simulink library "ddm"  (R2021b)
settings: Solver=VariableStepAuto  StartTime=0.0  StopTime=10.0  RelTol=1e-3
undefined symbols (not defined in the file or in its folder): ENUM_ADASACCSTA_ERROR, ENUM_ADASACCSTA_OFF, ENUM_ADASACCSTA_STANDBY, ENUM_ADASISASTA_OFF, ENUM_ALLOWMOV_ALLOWREADY, ENUM_APS, ENUM_BRKSTA_ERROR, ENUM_BRKSTA_OFF, ENUM_BRKSTA_ON, ENUM_BRKSW_INVALID, ENUM_BRKSW_OFF, ENUM_BRKSW_ON, ENUM_CHGPREACTERRSTA_OBCPRE, ENUM_DCDCFAULTSTA_ANYFAULTLV1, ENUM_DCDCFAULTSTA_ANYFAULTLV2, ENUM_DRIVETRAIN_AWD, ENUM_DRIVETRAIN_FWD, ENUM_DRIVETRAIN_RWD, ENUM_DRSEATSTA_INVALID, ENUM_EDUDRTSTA_NORMAL, ENUM_EPBSTA_APPLIED, ENUM_EPBSTA_RELEASED, ENUM_HVBATTREADYPRE_READY, ENUM_MCUWARN_LV0, ENUM_MCUWARN_LV1, ENUM_MCUWARN_LV2, ENUM_MCUWARN_LV3, ENUM_MCUWARN_NOERROR, ENUM_OBCFAULTSTA_ANYFAULT, ENUM_PAS_R2F2, ENUM_PDFAULT_BATTPDFAIL, ENUM_PDFAULT_DCDCDISABLE, ENUM_PDFAULT_MCUDISABLE, ENUM_PDFAULT_MCUDISCHRG, ENUM_POWERSTA_OFF, ENUM_POWERSTA_ON, ENUM_POWERSTA_READY, ENUM_POWERSTA_STANDBY, ENUM_PRESSINDI_LOW, ENUM_PUFAULT_BATTUPFAIL, ENUM_PUFAULT_DCDCENABLEFAIL, ENUM_PUFAULT_PRECHRGCHKFAIL, ENUM_PUFAULT_SAFETYCHKFAIL, ENUM_PUSTATE_COMPLETED, ENUM_PWRSTASW_OFF, ENUM_PWRSTASW_OFFA, ENUM_PWRSTASW_OFFCHVCHRG, ENUM_PWRSTASW_OFFCLVCHRG, ENUM_PWRSTASW_ON, ENUM_PWRSTASW_ONHVCHRG, ENUM_PWRSTASW_READY, ENUM_PWRSTASW_STANDBY, ENUM_RANGESTA_12IN, ENUM_SHIFTCOMMAND_D, ENUM_SHIFTCOMMAND_N, ENUM_SHIFTCOMMAND_P, ENUM_SHIFTCOMMAND_R, ENUM_VEHMALFUNLV_2ND, ENUM_VEHMALFUNLV_3RD, ENUM_VEHMALFUNLV_4TH ... (+835)
libraries: hcu_lib x750, $bdroot x12, simulink x5
(part 14 of 28)

== system ddm/DDM/DDM/VMC_DDM/CCU Signal Error ==
  task_time_s : Inport
  VDDM_C3CCU2LCCFS_flg : Inport  Port=2
  VDDM_C3CCU2RCCFS_flg : Inport  Port=3
  VDDM_C3CCU2CSCFS_flg : Inport  Port=4
  No_CAN_BUS_OFF : Inport  Port=5
  VPMM_PowerSta_enum : Inport  Port=6
  VINP_DCDCFaultSta_enum : Inport  Port=7
  DTC_clear_request : Inport  Port=8
  "CCU Signal Error " : Subsystem
  From5 : From  Commented=on  GotoTag=VDDM_CCUSigErrDFS_flg
  Terminator : Terminator
  VDDM_CCUSigErrCFS_flg : Outport
  VDDM_CCUSigErrDetDTC_raw32 : Outport  Port=2
  wires:
  [VDDM_CCUSigErrDetDTC_raw32] -> VDDM_CCUSigErrDetDTC_raw32/1
  "CCU Signal Error "/2(VDDM_CCUSigErrDetDTC_raw32) -> [VDDM_CCUSigErrDetDTC_raw32]
  [task_time_s] -> "CCU Signal Error "/1(task_time_s)
  task_time_s/1 -> [task_time_s]  "task_time_s"
  [DTC_clear_request] -> "CCU Signal Error "/8(DTC_clear_request)
  [VINP_DCDCFaultSta_enum] -> "CCU Signal Error "/7(VINP_DCDCFaultSta_enum)
  [VPMM_PowerSta_enum] -> "CCU Signal Error "/6(VPMM_PowerSta_enum)
  [No_CAN_BUS_OFF] -> "CCU Signal Error "/5(No_CAN_BUS_OFF)
  [VDDM_C3CCU2CSCFS_flg] -> "CCU Signal Error "/4(VDDM_C3CCU2CSCFS_flg)
  [VDDM_C3CCU2RCCFS_flg] -> "CCU Signal Error "/3(VDDM_C3CCU2RCCFS_flg)
  [VDDM_C3CCU2LCCFS_flg] -> "CCU Signal Error "/2(VDDM_C3CCU2LCCFS_flg)
  VINP_DCDCFaultSta_enum/1 -> [VINP_DCDCFaultSta_enum]
  VDDM_C3CCU2LCCFS_flg/1 -> [VDDM_C3CCU2LCCFS_flg]
  No_CAN_BUS_OFF/1 -> [No_CAN_BUS_OFF]
  VPMM_PowerSta_enum/1 -> [VPMM_PowerSta_enum]
  DTC_clear_request/1 -> [DTC_clear_request]
  "CCU Signal Error "/1(VDDM_CCUSigErrCFS_flg) -> [VDDM_CCUSigErrCFS_flg]
  From5/1 -> Terminator/1
  [VDDM_CCUSigErrCFS_flg] -> VDDM_CCUSigErrCFS_flg/1
  VDDM_C3CCU2RCCFS_flg/1 -> [VDDM_C3CCU2RCCFS_flg]
  VDDM_C3CCU2CSCFS_flg/1 -> [VDDM_C3CCU2CSCFS_flg]

== system ddm/DDM/DDM/VMC_DDM/FCM2 ==
  task_time_s : Inport
  VDDM_FCM2NoCom_flg : Inport  Port=2
  VDDM_FCM2RCErr_flg : Inport  Port=3
  VDDM_FCM2CSErr_flg : Inport  Port=4
  No_CAN_BUS_OFF : Inport  Port=5
  VPMM_PowerSta_enum : Inport  Port=6
  VINP_ADASACCSta_enum : Inport  Port=7
  DTC_clear_request : Inport  Port=8
  Constant18 : Constant  Commented=on  Value=TRUE
  Constant21 : Constant  Commented=on  Value=FALSE
  "FCM2 Checksum Error " : Subsystem
  FCM2 Lost Com : Subsystem
  "FCM2 Rolling Count Error " : Subsystem
  From15 : From  Commented=on  GotoTag=VDDM_FCM2NoComCFS_flg
  From16 : From  Commented=on  GotoTag=VDDM_FCM2RCErrCFS_flg
  From17 : From  Commented=on  GotoTag=VDDM_FCM2CSErrCFS_flg
  From30 : From  Commented=on  GotoTag=VDDM_VCUACCErr_flg
  Goto11 : Goto  Commented=on  GotoTag=VDDM_VCUACCErr_flg
  Logical Operator2 : Logic  Commented=on  Operator=OR  Inputs=3  AllPortsSameDT=off  OutDataTypeStr=boolean
  Switch : Switch  Commented=on  Criteria=u2 ~= 0
  Terminator : Terminator
  VDDM_FCM2NoComDFS_flg : Outport
  VDDM_FCM2NoComCFS_flg : Outport  Port=2
  VDDM_FCM2RCErrDFS_flg : Outport  Port=3
  VDDM_FCM2RCErrCFS_flg : Outport  Port=4
  VDDM_FCM2CSErrDFS_flg : Outport  Port=5
  VDDM_FCM2CSErrCFS_flg : Outport  Port=6
  VDDM_FCM2NoComDTC_raw32 : Outport  Port=7
  VDDM_FCM2RCErrDTC_raw32 : Outport  Port=8
  VDDM_FCM2CSErrDTC_raw32 : Outport  Port=9
  wires:
  [VDDM_FCM2CSErrDTC_raw32] -> VDDM_FCM2CSErrDTC_raw32/1
  [VDDM_FCM2RCErrDTC_raw32] -> VDDM_FCM2RCErrDTC_raw32/1
  [VDDM_FCM2NoComDTC_raw32] -> VDDM_FCM2NoComDTC_raw32/1
  "FCM2 Checksum Error "/3(VDDM_FCM2CSErrDTC_raw32) -> [VDDM_FCM2CSErrDTC_raw32]
  "FCM2 Rolling Count Error "/3(VDDM_FCM2RCErrDTC_raw32) -> [VDDM_FCM2RCErrDTC_raw32]
  FCM2 Lost Com/3(VDDM_FCM2NoComDTC_raw32) -> [VDDM_FCM2NoComDTC_raw32]
  "FCM2 Checksum Error "/2(VDDM_FCM2CSErrCFS_flg) -> [VDDM_FCM2CSErrCFS_flg]
  "FCM2 Checksum Error "/1(VDDM_FCM2CSErrDFS_flg) -> [VDDM_FCM2CSErrDFS_flg]
  [VDDM_FCM2NoComCFS_flg] -> "FCM2 Checksum Error "/4(VDDM_FCM2NoComCFS_flg)
  [VDDM_FCM2CSErr_flg] -> "FCM2 Checksum Error "/2(VDDM_FCM2CSErr_flg)
  [No_CAN_BUS_OFF] -> "FCM2 Checksum Error "/3(No_CAN_BUS_OFF)
  [VPMM_PowerSta_enum] -> "FCM2 Checksum Error "/5(VPMM_PowerSta_enum)
  [VINP_ADASACCSta_enum] -> "FCM2 Checksum Error "/6(VINP_ADASACCSta_enum)
  [DTC_clear_request] -> "FCM2 Checksum Error "/7(DTC_clear_request)
  [task_time_s] -> "FCM2 Checksum Error "/1(task_time_s)
  [task_time_s] -> "FCM2 Rolling Count Error "/1(task_time_s)
  task_time_s/1 -> [task_time_s]  "task_time_s"
  [task_time_s] -> FCM2 Lost Com/1(task_time_s)
  Logical Operator2/1 -> Switch/2
  From17/1 -> Logical Operator2/3
  From16/1 -> Logical Operator2/2
  From15/1 -> Logical Operator2/1
  Constant21/1 -> Switch/3
  Constant18/1 -> Switch/1
  VDDM_FCM2CSErr_flg/1 -> [VDDM_FCM2CSErr_flg]
  VDDM_FCM2RCErr_flg/1 -> [VDDM_FCM2RCErr_flg]
  From30/1 -> Terminator/1
  Switch/1 -> Goto11/1
  [VDDM_FCM2RCErrDFS_flg] -> VDDM_FCM2RCErrDFS_flg/1
  [VDDM_FCM2RCErrCFS_flg] -> VDDM_FCM2RCErrCFS_flg/1
  [VDDM_FCM2CSErrCFS_flg] -> VDDM_FCM2CSErrCFS_flg/1
  [VDDM_FCM2CSErrDFS_flg] -> VDDM_FCM2CSErrDFS_flg/1
  [VDDM_FCM2NoComCFS_flg] -> VDDM_FCM2NoComCFS_flg/1
  "FCM2 Rolling Count Error "/2(VDDM_FCM2RCErrCFS_flg) -> [VDDM_FCM2RCErrCFS_flg]
  "FCM2 Rolling Count Error "/1(VDDM_FCM2RCErrDFS_flg) -> [VDDM_FCM2RCErrDFS_flg]
  [DTC_clear_request] -> "FCM2 Rolling Count Error "/7(DTC_clear_request)
  [VINP_ADASACCSta_enum] -> "FCM2 Rolling Count Error "/6(VINP_ADASACCSta_enum)
  [VPMM_PowerSta_enum] -> "FCM2 Rolling Count Error "/5(VPMM_PowerSta_enum)
  [No_CAN_BUS_OFF] -> "FCM2 Rolling Count Error "/3(No_CAN_BUS_OFF)
  [VDDM_FCM2RCErr_flg] -> "FCM2 Rolling Count Error "/2(VDDM_FCM2RCErr_flg)
  [VDDM_FCM2NoComCFS_flg] -> "FCM2 Rolling Count Error "/4(VDDM_FCM2NoComCFS_flg)
  [VDDM_FCM2NoComDFS_flg] -> VDDM_FCM2NoComDFS_flg/1
  FCM2 Lost Com/1(VDDM_FCM2NoComDFS_flg) -> [VDDM_FCM2NoComDFS_flg]
  FCM2 Lost Com/2(VDDM_FCM2NoComCFS_flg) -> [VDDM_FCM2NoComCFS_flg]
  [DTC_clear_request] -> FCM2 Lost Com/6(DTC_clear_request)
  [VINP_ADASACCSta_enum] -> FCM2 Lost Com/5(VINP_ADASACCSta_enum)
  [VPMM_PowerSta_enum] -> FCM2 Lost Com/4(VPMM_PowerSta_enum)
  [No_CAN_BUS_OFF] -> FCM2 Lost Com/3(No_CAN_BUS_OFF)
  DTC_clear_request/1 -> [DTC_clear_request]
  VINP_ADASACCSta_enum/1 -> [VINP_ADASACCSta_enum]
  VPMM_PowerSta_enum/1 -> [VPMM_PowerSta_enum]
  No_CAN_BUS_OFF/1 -> [No_CAN_BUS_OFF]
  [VDDM_FCM2NoCom_flg] -> FCM2 Lost Com/2(VDDM_FCM2NoCom_flg)
  VDDM_FCM2NoCom_flg/1 -> [VDDM_FCM2NoCom_flg]

== system ddm/DDM/DDM/VMC_DDM/FCM3 ==
  task_time_s : Inport
  VDDM_FCM3NoCom_flg : Inport  Port=2
  VDDM_FCM3RCErr_flg : Inport  Port=3
  VDDM_FCM3CSErr_flg : Inport  Port=4
  No_CAN_BUS_OFF : Inport  Port=5
  VPMM_PowerSta_enum : Inport  Port=6
  VINP_ADASACCSta_enum : Inport  Port=7
  VINP_ADASISASta_enum : Inport  Port=8
  DTC_clear_request : Inport  Port=9
  Constant18 : Constant  Commented=on  Value=TRUE
  Constant21 : Constant  Commented=on  Value=FALSE
  "FCM3 Checksum Error " : Subsystem
  FCM3 Lost Com : Subsystem
  "FCM3 Rolling Count Error " : Subsystem
  From15 : From  Commented=on  GotoTag=VDDM_FCM3NoComCFS_flg
  From16 : From  Commented=on  GotoTag=VDDM_FCM3RCErrCFS_flg
  From17 : From  Commented=on  GotoTag=VDDM_FCM3CSErrCFS_flg
  From23 : From  Commented=on  GotoTag=VDDM_VCUISAErr_flg
  Goto11 : Goto  Commented=on  GotoTag=VDDM_VCUISAErr_flg
  Logical Operator2 : Logic  Commented=on  Operator=OR  Inputs=3  AllPortsSameDT=off  OutDataTypeStr=boolean
  Switch : Switch  Commented=on  Criteria=u2 ~= 0
  Terminator : Terminator
  VDDM_FCM3NoComDFS_flg : Outport
  VDDM_FCM3NoComCFS_flg : Outport  Port=2
  VDDM_FCM3RCErrDFS_flg : Outport  Port=3
  VDDM_FCM3RCErrCFS_flg : Outport  Port=4
  VDDM_FCM3CSErrDFS_flg : Outport  Port=5
  VDDM_FCM3CSErrCFS_flg : Outport  Port=6
  VDDM_FCM3NoComDTC_raw32 : Outport  Port=7
  VDDM_FCM3RCErrDTC_raw32 : Outport  Port=8
  VDDM_FCM3CSErrDTC_raw32 : Outport  Port=9
  wires:
  [VDDM_FCM3CSErrDTC_raw32] -> VDDM_FCM3CSErrDTC_raw32/1
  [VDDM_FCM3RCErrDTC_raw32] -> VDDM_FCM3RCErrDTC_raw32/1
  [VDDM_FCM3NoComDTC_raw32] -> VDDM_FCM3NoComDTC_raw32/1
  "FCM3 Checksum Error "/3(VDDM_FCM3CSErrDTC_raw32) -> [VDDM_FCM3CSErrDTC_raw32]
  "FCM3 Rolling Count Error "/3(VDDM_FCM3RCErrDTC_raw32) -> [VDDM_FCM3RCErrDTC_raw32]
  FCM3 Lost Com/3(VDDM_FCM3NoComDTC_raw32) -> [VDDM_FCM3NoComDTC_raw32]
  [VINP_ADASISASta_enum] -> "FCM3 Checksum Error "/7(VINP_ADASISASta_enum)
  [VINP_ADASISASta_enum] -> "FCM3 Rolling Count Error "/7(VINP_ADASISASta_enum)
  VINP_ADASISASta_enum/1 -> [VINP_ADASISASta_enum]
  [VINP_ADASISASta_enum] -> FCM3 Lost Com/6(VINP_ADASISASta_enum)
  "FCM3 Checksum Error "/2(VDDM_FCM3CSErrCFS_flg) -> [VDDM_FCM3CSErrCFS_flg]
  "FCM3 Checksum Error "/1(VDDM_FCM3CSErrDFS_flg) -> [VDDM_FCM3CSErrDFS_flg]
  [VDDM_FCM3NoComCFS_flg] -> "FCM3 Checksum Error "/4(VDDM_FCM3NoComCFS_flg)
  [VDDM_FCM3CSErr_flg] -> "FCM3 Checksum Error "/2(VDDM_FCM3CSErr_flg)
  [No_CAN_BUS_OFF] -> "FCM3 Checksum Error "/3(No_CAN_BUS_OFF)
  [VPMM_PowerSta_enum] -> "FCM3 Checksum Error "/5(VPMM_PowerSta_enum)
  [VINP_ADASACCSta_enum] -> "FCM3 Checksum Error "/6(VINP_ADASACCSta_enum)
  [DTC_clear_request] -> "FCM3 Checksum Error "/8(DTC_clear_request)
  [task_time_s] -> "FCM3 Checksum Error "/1(task_time_s)
  [task_time_s] -> "FCM3 Rolling Count Error "/1(task_time_s)
  task_time_s/1 -> [task_time_s]  "task_time_s"
  [task_time_s] -> FCM3 Lost Com/1(task_time_s)
  Logical Operator2/1 -> Switch/2
  From17/1 -> Logical Operator2/3
  From16/1 -> Logical Operator2/2
  From15/1 -> Logical Operator2/1
  Constant21/1 -> Switch/3
  Constant18/1 -> Switch/1
  VDDM_FCM3CSErr_flg/1 -> [VDDM_FCM3CSErr_flg]
  VDDM_FCM3RCErr_flg/1 -> [VDDM_FCM3RCErr_flg]
  From23/1 -> Terminator/1
  Switch/1 -> Goto11/1
  [VDDM_FCM3RCErrDFS_flg] -> VDDM_FCM3RCErrDFS_flg/1
  [VDDM_FCM3RCErrCFS_flg] -> VDDM_FCM3RCErrCFS_flg/1
  [VDDM_FCM3CSErrCFS_flg] -> VDDM_FCM3CSErrCFS_flg/1
  [VDDM_FCM3CSErrDFS_flg] -> VDDM_FCM3CSErrDFS_flg/1
  [VDDM_FCM3NoComCFS_flg] -> VDDM_FCM3NoComCFS_flg/1
  "FCM3 Rolling Count Error "/2(VDDM_FCM3RCErrCFS_flg) -> [VDDM_FCM3RCErrCFS_flg]
  "FCM3 Rolling Count Error "/1(VDDM_FCM3RCErrDFS_flg) -> [VDDM_FCM3RCErrDFS_flg]
  [DTC_clear_request] -> "FCM3 Rolling Count Error "/8(DTC_clear_request)
  [VINP_ADASACCSta_enum] -> "FCM3 Rolling Count Error "/6(VINP_ADASACCSta_enum)
  [VPMM_PowerSta_enum] -> "FCM3 Rolling Count Error "/5(VPMM_PowerSta_enum)
  [No_CAN_BUS_OFF] -> "FCM3 Rolling Count Error "/3(No_CAN_BUS_OFF)
  [VDDM_FCM3RCErr_flg] -> "FCM3 Rolling Count Error "/2(VDDM_FCM3RCErr_flg)
  [VDDM_FCM3NoComCFS_flg] -> "FCM3 Rolling Count Error "/4(VDDM_FCM3NoComCFS_flg)
  [VDDM_FCM3NoComDFS_flg] -> VDDM_FCM3NoComDFS_flg/1
  FCM3 Lost Com/1(VDDM_FCM3NoComDFS_flg) -> [VDDM_FCM3NoComDFS_flg]
  FCM3 Lost Com/2(VDDM_FCM3NoComCFS_flg) -> [VDDM_FCM3NoComCFS_flg]
  [DTC_clear_request] -> FCM3 Lost Com/7(DTC_clear_request)
  [VINP_ADASACCSta_enum] -> FCM3 Lost Com/5(VINP_ADASACCSta_enum)
  [VPMM_PowerSta_enum] -> FCM3 Lost Com/4(VPMM_PowerSta_enum)
  [No_CAN_BUS_OFF] -> FCM3 Lost Com/3(No_CAN_BUS_OFF)
  DTC_clear_request/1 -> [DTC_clear_request]
  VINP_ADASACCSta_enum/1 -> [VINP_ADASACCSta_enum]
  VPMM_PowerSta_enum/1 -> [VPMM_PowerSta_enum]
  No_CAN_BUS_OFF/1 -> [No_CAN_BUS_OFF]
  [VDDM_FCM3NoCom_flg] -> FCM3 Lost Com/2(VDDM_FCM3NoCom_flg)
  VDDM_FCM3NoCom_flg/1 -> [VDDM_FCM3NoCom_flg]

== system ddm/DDM/DDM/VMC_DDM/FCM4 ==
  task_time_s : Inport
  VDDM_FCM4NoCom_flg : Inport  Port=2
  VDDM_FCM4CSErr_flg : Inport  Port=3
  No_CAN_BUS_OFF : Inport  Port=4
  VPMM_PowerSta_enum : Inport  Port=5
  VINP_ADASACCSta_enum : Inport  Port=6
  DTC_clear_request : Inport  Port=7
  Constant18 : Constant  Commented=on  Value=TRUE
  Constant21 : Constant  Commented=on  Value=FALSE
  "FCM4 Checksum Error " : Subsystem
  FCM4 Lost Com : Subsystem
  "FCM4 Rolling Count Error " : Subsystem  Commented=on
  From10 : From  Commented=on  GotoTag=VINP_ADASACCSta_enum
  From11 : From  Commented=on  GotoTag=DTC_clear_request
  From15 : From  Commented=on  GotoTag=VDDM_FCM4NoComCFS_flg
  From16 : From  Commented=on  GotoTag=VDDM_FCM4RCErrCFS_flg
  From17 : From  Commented=on  GotoTag=VDDM_FCM4CSErrCFS_flg
  From19 : From  Commented=on  GotoTag=task_time_s
  From21 : From  Commented=on  GotoTag=VDDM_FCM4RCErrCFS_flg
  From22 : From  Commented=on  GotoTag=VDDM_FCM4RCErrDFS_flg
  From30 : From  Commented=on  GotoTag=VDDM_VCUACCErr_flg
  From6 : From  Commented=on  GotoTag=VDDM_FCM4NoComCFS_flg
  From7 : From  Commented=on  GotoTag=VDDM_FCM4RCErr_flg
  From8 : From  Commented=on  GotoTag=No_CAN_BUS_OFF
  From9 : From  Commented=on  GotoTag=VPMM_PowerSta_enum
  Goto11 : Goto  Commented=on  GotoTag=VDDM_VCUACCErr_flg
  Goto12 : Goto  Commented=on  GotoTag=VDDM_FCM4RCErr_flg
  Goto7 : Goto  Commented=on  GotoTag=VDDM_FCM4RCErrCFS_flg
  Goto8 : Goto  Commented=on  GotoTag=VDDM_FCM4RCErrDFS_flg
  Ground : Ground
  Logical Operator2 : Logic  Commented=on  Operator=OR  Inputs=3  AllPortsSameDT=off  OutDataTypeStr=boolean
  Switch : Switch  Commented=on  Criteria=u2 ~= 0
  Terminator : Terminator
  Terminator1 : Terminator
  Terminator2 : Terminator
  VDDM_FCM4NoComDFS_flg : Outport
  VDDM_FCM4NoComCFS_flg : Outport  Port=2
  VDDM_FCM4CSErrDFS_flg : Outport  Port=3
  VDDM_FCM4CSErrCFS_flg : Outport  Port=4
  VDDM_FCM4NoComDTC_raw32 : Outport  Port=5
  VDDM_FCM4CSErrDTC_raw32 : Outport  Port=6
  wires:
  [VDDM_FCM4CSErrDTC_raw32] -> VDDM_FCM4CSErrDTC_raw32/1
  [VDDM_FCM4NoComDTC_raw32] -> VDDM_FCM4NoComDTC_raw32/1
  "FCM4 Checksum Error "/3(VDDM_FCM4CSErrDTC_raw32) -> [VDDM_FCM4CSErrDTC_raw32]
  FCM4 Lost Com/3(VDDM_FCM4NoComDTC_raw32) -> [VDDM_FCM4NoComDTC_raw32]
  "FCM4 Checksum Error "/2(VDDM_FCM4CSErrCFS_flg) -> [VDDM_FCM4CSErrCFS_flg]
  "FCM4 Checksum Error "/1(VDDM_FCM4CSErrDFS_flg) -> [VDDM_FCM4CSErrDFS_flg]
  [VDDM_FCM4NoComCFS_flg] -> "FCM4 Checksum Error "/4(VDDM_FCM4NoComCFS_flg)
  [VDDM_FCM4CSErr_flg] -> "FCM4 Checksum Error "/2(VDDM_FCM4CSErr_flg)
  [No_CAN_BUS_OFF] -> "FCM4 Checksum Error "/3(No_CAN_BUS_OFF)
  [VPMM_PowerSta_enum] -> "FCM4 Checksum Error "/5(VPMM_PowerSta_enum)
  [VINP_ADASACCSta_enum] -> "FCM4 Checksum Error "/6(VINP_ADASACCSta_enum)
  [DTC_clear_request] -> "FCM4 Checksum Error "/7(DTC_clear_request)
  [task_time_s] -> "FCM4 Checksum Error "/1(task_time_s)
  From19/1 -> "FCM4 Rolling Count Error "/1(task_time_s)
  task_time_s/1 -> [task_time_s]  "task_time_s"
  [task_time_s] -> FCM4 Lost Com/1(task_time_s)
  Logical Operator2/1 -> Switch/2
  From17/1 -> Logical Operator2/3
  From16/1 -> Logical Operator2/2
  From15/1 -> Logical Operator2/1
  Constant21/1 -> Switch/3
  Constant18/1 -> Switch/1
  VDDM_FCM4CSErr_flg/1 -> [VDDM_FCM4CSErr_flg]
  Ground/1 -> Goto12/1
  From30/1 -> Terminator2/1
  Switch/1 -> Goto11/1
  From22/1 -> Terminator/1
  From21/1 -> Terminator1/1
  [VDDM_FCM4CSErrCFS_flg] -> VDDM_FCM4CSErrCFS_flg/1
  [VDDM_FCM4CSErrDFS_flg] -> VDDM_FCM4CSErrDFS_flg/1
  [VDDM_FCM4NoComCFS_flg] -> VDDM_FCM4NoComCFS_flg/1
  "FCM4 Rolling Count Error "/2(VDDM_FCM4RCErrCFS_flg) -> Goto7/1
  "FCM4 Rolling Count Error "/1(VDDM_FCM4RCErrDFS_flg) -> Goto8/1
  From11/1 -> "FCM4 Rolling Count Error "/7(DTC_clear_request)
  From10/1 -> "FCM4 Rolling Count Error "/6(VINP_ADASACCSta_enum)
  From9/1 -> "FCM4 Rolling Count Error "/5(VPMM_PowerSta_enum)
  From8/1 -> "FCM4 Rolling Count Error "/3(No_CAN_BUS_OFF)
  From7/1 -> "FCM4 Rolling Count Error "/2(VDDM_FCM4RCErr_flg)
  From6/1 -> "FCM4 Rolling Count Error "/4(VDDM_FCM4NoComCFS_flg)
  [VDDM_FCM4NoComDFS_flg] -> VDDM_FCM4NoComDFS_flg/1
  FCM4 Lost Com/1(VDDM_FCM4NoComDFS_flg) -> [VDDM_FCM4NoComDFS_flg]
  FCM4 Lost Com/2(VDDM_FCM4NoComCFS_flg) -> [VDDM_FCM4NoComCFS_flg]
  [DTC_clear_request] -> FCM4 Lost Com/6(DTC_clear_request)
  [VINP_ADASACCSta_enum] -> FCM4 Lost Com/5(VINP_ADASACCSta_enum)
  [VPMM_PowerSta_enum] -> FCM4 Lost Com/4(VPMM_PowerSta_enum)
  [No_CAN_BUS_OFF] -> FCM4 Lost Com/3(No_CAN_BUS_OFF)
  DTC_clear_request/1 -> [DTC_clear_request]
  VINP_ADASACCSta_enum/1 -> [VINP_ADASACCSta_enum]
  VPMM_PowerSta_enum/1 -> [VPMM_PowerSta_enum]
  No_CAN_BUS_OFF/1 -> [No_CAN_BUS_OFF]
  [VDDM_FCM4NoCom_flg] -> FCM4 Lost Com/2(VDDM_FCM4NoCom_flg)
  VDDM_FCM4NoCom_flg/1 -> [VDDM_FCM4NoCom_flg]

== system ddm/DDM/DDM/VMC_DDM/FCM5 ==
  task_time_s : Inport
  VDDM_FCM5NoCom_flg : Inport  Port=2
  VDDM_FCM5CSErr_flg : Inport  Port=3
  No_CAN_BUS_OFF : Inport  Port=4
  VPMM_PowerSta_enum : Inport  Port=5
  VINP_ADASISASta_enum : Inport  Port=6
  DTC_clear_request : Inport  Port=7
  Constant18 : Constant  Commented=on  Value=TRUE
  Constant21 : Constant  Commented=on  Value=FALSE
  "FCM5 Checksum Error " : Subsystem
  FCM5 Lost Com : Subsystem
  "FCM5 Rolling Count Error " : Subsystem  Commented=on
  From11 : From  Commented=on  GotoTag=DTC_clear_request
  From15 : From  Commented=on  GotoTag=VDDM_FCM5NoComCFS_flg
  From16 : From  Commented=on  GotoTag=VDDM_FCM5RCErrCFS_flg
  From17 : From  Commented=on  GotoTag=VDDM_FCM5CSErrCFS_flg
  From19 : From  Commented=on  GotoTag=task_time_s
  From21 : From  Commented=on  GotoTag=VDDM_FCM5RCErrCFS_flg
  From22 : From  Commented=on  GotoTag=VDDM_FCM5RCErrDFS_flg
  From23 : From  Commented=on  GotoTag=VDDM_VCUISAErr_flg
  From31 : From  Commented=on  GotoTag=VINP_ADASISASta_enum
  From6 : From  Commented=on  GotoTag=VDDM_FCM5NoComCFS_flg
  From7 : From  Commented=on  GotoTag=VDDM_FCM5RCErr_flg
  From8 : From  Commented=on  GotoTag=No_CAN_BUS_OFF
  From9 : From  Commented=on  GotoTag=VPMM_PowerSta_enum
  Goto11 : Goto  Commented=on  GotoTag=VDDM_VCUISAErr_flg
  Goto12 : Goto  Commented=on  GotoTag=VDDM_FCM5RCErr_flg
  Goto7 : Goto  Commented=on  GotoTag=VDDM_FCM5RCErrCFS_flg
  Goto8 : Goto  Commented=on  GotoTag=VDDM_FCM5RCErrDFS_flg
  Ground : Ground
  Logical Operator2 : Logic  Commented=on  Operator=OR  Inputs=3  AllPortsSameDT=off  OutDataTypeStr=boolean
  Switch : Switch  Commented=on  Criteria=u2 ~= 0
  Terminator : Terminator
  Terminator1 : Terminator
  Terminator2 : Terminator
  VDDM_FCM5NoComDFS_flg : Outport
  VDDM_FCM5NoComCFS_flg : Outport  Port=2
  VDDM_FCM5CSErrDFS_flg : Outport  Port=3
  VDDM_FCM5CSErrCFS_flg : Outport  Port=4
  VDDM_FCM5NoComDTC_raw32 : Outport  Port=5
  VDDM_FCM5CSErrDTC_raw32 : Outport  Port=6
  wires:
  [VDDM_FCM5CSErrDTC_raw32] -> VDDM_FCM5CSErrDTC_raw32/1
  [VDDM_FCM5NoComDTC_raw32] -> VDDM_FCM5NoComDTC_raw32/1
  "FCM5 Checksum Error "/3(VDDM_FCM5CSErrDTC_raw32) -> [VDDM_FCM5CSErrDTC_raw32]
  FCM5 Lost Com/3(VDDM_FCM5NoComDTC_raw32) -> [VDDM_FCM5NoComDTC_raw32]
  [VINP_ADASISASta_enum] -> "FCM5 Checksum Error "/6(VINP_ADASISASta_enum)
  From31/1 -> "FCM5 Rolling Count Error "/6(VINP_ADASISASta_enum)
  VINP_ADASISASta_enum/1 -> [VINP_ADASISASta_enum]
  [VINP_ADASISASta_enum] -> FCM5 Lost Com/5(VINP_ADASISASta_enum)
  "FCM5 Checksum Error "/2(VDDM_FCM5CSErrCFS_flg) -> [VDDM_FCM5CSErrCFS_flg]
  "FCM5 Checksum Error "/1(VDDM_FCM5CSErrDFS_flg) -> [VDDM_FCM5CSErrDFS_flg]
  [VDDM_FCM5NoComCFS_flg] -> "FCM5 Checksum Error "/4(VDDM_FCM5NoComCFS_flg)
  [VDDM_FCM5CSErr_flg] -> "FCM5 Checksum Error "/2(VDDM_FCM5CSErr_flg)
  [No_CAN_BUS_OFF] -> "FCM5 Checksum Error "/3(No_CAN_BUS_OFF)
  [VPMM_PowerSta_enum] -> "FCM5 Checksum Error "/5(VPMM_PowerSta_enum)
  [DTC_clear_request] -> "FCM5 Checksum Error "/7(DTC_clear_request)
  [task_time_s] -> "FCM5 Checksum Error "/1(task_time_s)
  From19/1 -> "FCM5 Rolling Count Error "/1(task_time_s)
  task_time_s/1 -> [task_time_s]  "task_time_s"
  [task_time_s] -> FCM5 Lost Com/1(task_time_s)
  Logical Operator2/1 -> Switch/2
  From17/1 -> Logical Operator2/3
  From16/1 -> Logical Operator2/2
  From15/1 -> Logical Operator2/1
  Constant21/1 -> Switch/3
  Constant18/1 -> Switch/1
  VDDM_FCM5CSErr_flg/1 -> [VDDM_FCM5CSErr_flg]
  Ground/1 -> Goto12/1
  From23/1 -> Terminator2/1
  Switch/1 -> Goto11/1
  From22/1 -> Terminator/1
  From21/1 -> Terminator1/1
  [VDDM_FCM5CSErrCFS_flg] -> VDDM_FCM5CSErrCFS_flg/1
  [VDDM_FCM5CSErrDFS_flg] -> VDDM_FCM5CSErrDFS_flg/1
  [VDDM_FCM5NoComCFS_flg] -> VDDM_FCM5NoComCFS_flg/1
  "FCM5 Rolling Count Error "/2(VDDM_FCM5RCErrCFS_flg) -> Goto7/1
  "FCM5 Rolling Count Error "/1(VDDM_FCM5RCErrDFS_flg) -> Goto8/1
  From11/1 -> "FCM5 Rolling Count Error "/7(DTC_clear_request)
  From9/1 -> "FCM5 Rolling Count Error "/5(VPMM_PowerSta_enum)
  From8/1 -> "FCM5 Rolling Count Error "/3(No_CAN_BUS_OFF)
  From7/1 -> "FCM5 Rolling Count Error "/2(VDDM_FCM5RCErr_flg)
  From6/1 -> "FCM5 Rolling Count Error "/4(VDDM_FCM5NoComCFS_flg)
  [VDDM_FCM5NoComDFS_flg] -> VDDM_FCM5NoComDFS_flg/1
  FCM5 Lost Com/1(VDDM_FCM5NoComDFS_flg) -> [VDDM_FCM5NoComDFS_flg]
  FCM5 Lost Com/2(VDDM_FCM5NoComCFS_flg) -> [VDDM_FCM5NoComCFS_flg]
  [DTC_clear_request] -> FCM5 Lost Com/6(DTC_clear_request)
  [VPMM_PowerSta_enum] -> FCM5 Lost Com/4(VPMM_PowerSta_enum)
  [No_CAN_BUS_OFF] -> FCM5 Lost Com/3(No_CAN_BUS_OFF)
  DTC_clear_request/1 -> [DTC_clear_request]
  VPMM_PowerSta_enum/1 -> [VPMM_PowerSta_enum]
  No_CAN_BUS_OFF/1 -> [No_CAN_BUS_OFF]
  [VDDM_FCM5NoCom_flg] -> FCM5 Lost Com/2(VDDM_FCM5NoCom_flg)
  VDDM_FCM5NoCom_flg/1 -> [VDDM_FCM5NoCom_flg]

== system ddm/DDM/DDM/VMC_DDM/FCMACC Signal Error ==
  task_time_s : Inport
  VDDM_FCM4NoComCFS_flg : Inport  Port=2
  VDDM_FCM4CSErrCFS_flg : Inport  Port=3
  No_CAN_BUS_OFF : Inport  Port=4
  VPMM_PowerSta_enum : Inport  Port=5
  VINP_ADASACCSta_enum : Inport  Port=6
  DTC_clear_request : Inport  Port=7
  "FCMACC Signal Error " : Subsystem
  From5 : From  Commented=on  GotoTag=VDDM_FCMACCSigErrDFS_flg
  Terminator : Terminator
  VDDM_FCMACCSigErrCFS_flg : Outport
  VDDM_FCMACCSigErrDetDTC_raw32 : Outport  Port=2
  wires:
  [VDDM_FCMACCSigErrDetDTC_raw32] -> VDDM_FCMACCSigErrDetDTC_raw32/1
  "FCMACC Signal Error "/2(VDDM_FCMACCSigErrDetDTC_raw32) -> [VDDM_FCMACCSigErrDetDTC_raw32]
  [VINP_ADASACCSta_enum] -> "FCMACC Signal Error "/6(VINP_ADASACCSta_enum)
  VINP_ADASACCSta_enum/1 -> [VINP_ADASACCSta_enum]
  [VDDM_FCM4CSErrCFS_flg] -> "FCMACC Signal Error "/3(VDDM_FCM4CSErrCFS_flg)
  [VDDM_FCM4NoComCFS_flg] -> "FCMACC Signal Error "/2(VDDM_FCM4NoComCFS_flg)
  [task_time_s] -> "FCMACC Signal Error "/1(task_time_s)
  task_time_s/1 -> [task_time_s]  "task_time_s"
  [DTC_clear_request] -> "FCMACC Signal Error "/7(DTC_clear_request)
  [VPMM_PowerSta_enum] -> "FCMACC Signal Error "/5(VPMM_PowerSta_enum)
  [No_CAN_BUS_OFF] -> "FCMACC Signal Error "/4(No_CAN_BUS_OFF)
  VDDM_FCM4NoComCFS_flg/1 -> [VDDM_FCM4NoComCFS_flg]
  No_CAN_BUS_OFF/1 -> [No_CAN_BUS_OFF]
  VPMM_PowerSta_enum/1 -> [VPMM_PowerSta_enum]
  DTC_clear_request/1 -> [DTC_clear_request]
  "FCMACC Signal Error "/1(VDDM_FCMACCSigErrCFS_flg) -> [VDDM_FCMACCSigErrCFS_flg]
  From5/1 -> Terminator/1
  [VDDM_FCMACCSigErrCFS_flg] -> VDDM_FCMACCSigErrCFS_flg/1
  VDDM_FCM4CSErrCFS_flg/1 -> [VDDM_FCM4CSErrCFS_flg]

== system ddm/DDM/DDM/VMC_DDM/ISA Malfunction  ==
  task_time_s : Inport
  VDDM_BMSSigErrCFS_flg : Inport  Port=2
  VDDM_FrMCUSigErrCFS_flg : Inport  Port=3
  VDDM_RrMCUSigErrCFS_flg : Inport  Port=4
  VDDM_CCUSigErrCFS_flg : Inport  Port=5
  VDDM_FCM3NoComCFS_flg : Inport  Port=6
  VDDM_FCM3RCErrCFS_flg : Inport  Port=7
  VDDM_FCM3CSErrCFS_flg : Inport  Port=8
  VDDM_FCM5NoComCFS_flg : Inport  Port=9
  VDDM_FCM5CSErrCFS_flg : Inport  Port=10
  VDDM_ZoneSCPNoComCFS_flg : Inport  Port=11
  VDDM_MCUR1NoComCFS_flg : Inport  Port=12
  VDDM_MCUR1RCErrCFS_flg : Inport  Port=13
  VDDM_MCUR1CSErrCFS_flg : Inport  Port=14
  VDDM_MCUF1NoComCFS_flg : Inport  Port=15
  VDDM_MCUF1RCErrCFS_flg : Inport  Port=16
  VDDM_MCUF1CSErrCFS_flg : Inport  Port=17
  VDDM_ESC7NoComCFS_flg : Inport  Port=18
  VDDM_ESC7RCErrCFS_flg : Inport  Port=19
  VDDM_ESC7CSErrCFS_flg : Inport  Port=20
  VDDM_ESC1NoComCFS_flg : Inport  Port=21
  VDDM_ESC1RCErrCFS_flg : Inport  Port=22
  VDDM_ESC1CSErrCFS_flg : Inport  Port=23
  VDDM_ESC5NoComCFS_flg : Inport  Port=24
  VDDM_ESC5RCErrCFS_flg : Inport  Port=25
  VDDM_ESC5CSErrCFS_flg : Inport  Port=26
  No_CAN1_BUS_OFF : Inport  Port=27
  No_CAN3_BUS_OFF : Inport  Port=28
  No_CAN4_BUS_OFF : Inport  Port=29
  VPMM_PowerSta_enum : Inport  Port=30
  VINP_ZoneSpdCtrlMode_enum : Inport  Port=31
  DTC_clear_request : Inport  Port=32
  From5 : From  Commented=on  GotoTag=VDDM_ISAMalfuncDFS_flg
  ISA Malfunction : Subsystem
  Terminator : Terminator
  VDDM_ISAMalfuncCFS_flg : Outport
  VDDM_ISAMalfuncDetDTC_raw32 : Outport  Port=2
  wires:
  [VDDM_ISAMalfuncDetDTC_raw32] -> VDDM_ISAMalfuncDetDTC_raw32/1
  ISA Malfunction/2(VDDM_ISAMalfuncDetDTC_raw32) -> [VDDM_ISAMalfuncDetDTC_raw32]
  VDDM_FCM3NoComCFS_flg/1 -> [VDDM_FCM3NoComCFS_flg]
  VDDM_FCM5CSErrCFS_flg/1 -> [VDDM_FCM5CSErrCFS_flg]
  VDDM_FCM5NoComCFS_flg/1 -> [VDDM_FCM5NoComCFS_flg]
  VDDM_FCM3RCErrCFS_flg/1 -> [VDDM_FCM3RCErrCFS_flg]
  VDDM_FCM3CSErrCFS_flg/1 -> [VDDM_FCM3CSErrCFS_flg]
  [DTC_clear_request] -> ISA Malfunction/32(DTC_clear_request)
  [VINP_ZoneSpdCtrlMode_enum] -> ISA Malfunction/31(VINP_ZoneSpdCtrlMode_enum)
  [VPMM_PowerSta_enum] -> ISA Malfunction/30(VPMM_PowerSta_enum)
  [No_CAN4_BUS_OFF] -> ISA Malfunction/29(No_CAN4_BUS_OFF)
  [No_CAN3_BUS_OFF] -> ISA Malfunction/28(No_CAN3_BUS_OFF)
  [No_CAN1_BUS_OFF] -> ISA Malfunction/27(No_CAN1_BUS_OFF)
  [VDDM_ESC5CSErrCFS_flg] -> ISA Malfunction/26(VDDM_ESC5CSErrCFS_flg)
  [VDDM_ESC5RCErrCFS_flg] -> ISA Malfunction/25(VDDM_ESC5RCErrCFS_flg)
  [VDDM_ESC5NoComCFS_flg] -> ISA Malfunction/24(VDDM_ESC5NoComCFS_flg)
  [VDDM_ESC1CSErrCFS_flg] -> ISA Malfunction/23(VDDM_ESC1CSErrCFS_flg)
  [VDDM_ESC1RCErrCFS_flg] -> ISA Malfunction/22(VDDM_ESC1RCErrCFS_flg)
  [VDDM_ESC1NoComCFS_flg] -> ISA Malfunction/21(VDDM_ESC1NoComCFS_flg)
  [VDDM_ESC7CSErrCFS_flg] -> ISA Malfunction/20(VDDM_ESC7CSErrCFS_flg)
  [VDDM_ESC7RCErrCFS_flg] -> ISA Malfunction/19(VDDM_ESC7RCErrCFS_flg)
  [VDDM_ESC7NoComCFS_flg] -> ISA Malfunction/18(VDDM_ESC7NoComCFS_flg)
  [VDDM_MCUF1CSErrCFS_flg] -> ISA Malfunction/17(VDDM_MCUF1CSErrCFS_flg)
  [VDDM_MCUF1RCErrCFS_flg] -> ISA Malfunction/16(VDDM_MCUF1RCErrCFS_flg)
  [VDDM_MCUF1NoComCFS_flg] -> ISA Malfunction/15(VDDM_MCUF1NoComCFS_flg)
  [VDDM_MCUR1CSErrCFS_flg] -> ISA Malfunction/14(VDDM_MCUR1CSErrCFS_flg)
  [VDDM_MCUR1RCErrCFS_flg] -> ISA Malfunction/13(VDDM_MCUR1RCErrCFS_flg)
  [VDDM_MCUR1NoComCFS_flg] -> ISA Malfunction/12(VDDM_MCUR1NoComCFS_flg)
  [VDDM_ZoneSCPNoComCFS_flg] -> ISA Malfunction/11(VDDM_ZoneSCPNoComCFS_flg)
  [VDDM_FCM5CSErrCFS_flg] -> ISA Malfunction/10(VDDM_FCM5CSErrCFS_flg)
  [VDDM_FCM5NoComCFS_flg] -> ISA Malfunction/9(VDDM_FCM5NoComCFS_flg)
  [VDDM_FCM3CSErrCFS_flg] -> ISA Malfunction/8(VDDM_FCM3CSErrCFS_flg)
  [VDDM_FCM3RCErrCFS_flg] -> ISA Malfunction/7(VDDM_FCM3RCErrCFS_flg)
  [VDDM_FCM3NoComCFS_flg] -> ISA Malfunction/6(VDDM_FCM3NoComCFS_flg)
  [VDDM_CCUSigErrCFS_flg] -> ISA Malfunction/5(VDDM_CCUSigErrCFS_flg)
  [VDDM_RrMCUSigErrCFS_flg] -> ISA Malfunction/4(VDDM_RrMCUSigErrCFS_flg)
  [VDDM_FrMCUSigErrCFS_flg] -> ISA Malfunction/3(VDDM_FrMCUSigErrCFS_flg)
  [VDDM_BMSSigErrCFS_flg] -> ISA Malfunction/2(VDDM_BMSSigErrCFS_flg)
  [task_time_s] -> ISA Malfunction/1(task_time_s)
  DTC_clear_request/1 -> [DTC_clear_request]
  No_CAN4_BUS_OFF/1 -> [No_CAN4_BUS_OFF]
  No_CAN3_BUS_OFF/1 -> [No_CAN3_BUS_OFF]
  VDDM_ESC5NoComCFS_flg/1 -> [VDDM_ESC5NoComCFS_flg]
  VDDM_ESC5RCErrCFS_flg/1 -> [VDDM_ESC5RCErrCFS_flg]
  VDDM_ESC5CSErrCFS_flg/1 -> [VDDM_ESC5CSErrCFS_flg]
  VDDM_MCUR1CSErrCFS_flg/1 -> [VDDM_MCUR1CSErrCFS_flg]
  VDDM_MCUR1RCErrCFS_flg/1 -> [VDDM_MCUR1RCErrCFS_flg]
  VDDM_MCUR1NoComCFS_flg/1 -> [VDDM_MCUR1NoComCFS_flg]
  VDDM_MCUF1NoComCFS_flg/1 -> [VDDM_MCUF1NoComCFS_flg]
  VDDM_MCUF1RCErrCFS_flg/1 -> [VDDM_MCUF1RCErrCFS_flg]
  VDDM_MCUF1CSErrCFS_flg/1 -> [VDDM_MCUF1CSErrCFS_flg]
  VDDM_ESC1CSErrCFS_flg/1 -> [VDDM_ESC1CSErrCFS_flg]
  VDDM_ESC1RCErrCFS_flg/1 -> [VDDM_ESC1RCErrCFS_flg]
  VDDM_ESC1NoComCFS_flg/1 -> [VDDM_ESC1NoComCFS_flg]
  VDDM_ESC7NoComCFS_flg/1 -> [VDDM_ESC7NoComCFS_flg]
  VDDM_ESC7RCErrCFS_flg/1 -> [VDDM_ESC7RCErrCFS_flg]
  VDDM_ESC7CSErrCFS_flg/1 -> [VDDM_ESC7CSErrCFS_flg]
  VDDM_ZoneSCPNoComCFS_flg/1 -> [VDDM_ZoneSCPNoComCFS_flg]
  VDDM_CCUSigErrCFS_flg/1 -> [VDDM_CCUSigErrCFS_flg]
  VDDM_RrMCUSigErrCFS_flg/1 -> [VDDM_RrMCUSigErrCFS_flg]
  VDDM_FrMCUSigErrCFS_flg/1 -> [VDDM_FrMCUSigErrCFS_flg]
  task_time_s/1 -> [task_time_s]  "task_time_s"
  VINP_ZoneSpdCtrlMode_enum/1 -> [VINP_ZoneSpdCtrlMode_enum]
  No_CAN1_BUS_OFF/1 -> [No_CAN1_BUS_OFF]
  VPMM_PowerSta_enum/1 -> [VPMM_PowerSta_enum]
  ISA Malfunction/1(VDDM_ISAMalfuncCFS_flg) -> [VDDM_ISAMalfuncCFS_flg]
  From5/1 -> Terminator/1
  [VDDM_ISAMalfuncCFS_flg] -> VDDM_ISAMalfuncCFS_flg/1
  VDDM_BMSSigErrCFS_flg/1 -> [VDDM_BMSSigErrCFS_flg]

== system ddm/DDM/DDM/VMC_DDM/MCU_Fr Signal Error ==
  task_time_s : Inport
  VDDM_MCUF1NoComCFS_flg : Inport  Port=2
  VDDM_MCUF1RCErrCFS_flg : Inport  Port=3
  VDDM_MCUF1CSErrCFS_flg : Inport  Port=4
  No_CAN_BUS_OFF : Inport  Port=5
  VPMM_PowerSta_enum : Inport  Port=6
  VINP_MCUWarnF_enum : Inport  Port=7
  DTC_clear_request : Inport  Port=8
  From5 : From  Commented=on  GotoTag=VDDM_FrMCUSigErrDFS_flg
  "MCU_Fr Signal Error " : Subsystem
  Terminator : Terminator
  VDDM_FrMCUSigErrCFS_flg : Outport
  VDDM_FrMCUSigErrDetDTC_raw32 : Outport  Port=2
  wires:
  [VDDM_FrMCUSigErrDetDTC_raw32] -> VDDM_FrMCUSigErrDetDTC_raw32/1
  "MCU_Fr Signal Error "/2(VDDM_FrMCUSigErrDetDTC_raw32) -> [VDDM_FrMCUSigErrDetDTC_raw32]
  [task_time_s] -> "MCU_Fr Signal Error "/1(task_time_s)
  task_time_s/1 -> [task_time_s]  "task_time_s"
  [DTC_clear_request] -> "MCU_Fr Signal Error "/8(DTC_clear_request)
  [VINP_MCUWarnF_enum] -> "MCU_Fr Signal Error "/7(VINP_MCUWarnF_enum)
  [VPMM_PowerSta_enum] -> "MCU_Fr Signal Error "/6(VPMM_PowerSta_enum)
  [No_CAN_BUS_OFF] -> "MCU_Fr Signal Error "/5(No_CAN_BUS_OFF)
  [VDDM_MCUF1CSErrCFS_flg] -> "MCU_Fr Signal Error "/4(VDDM_MCUF1CSErrCFS_flg)
  [VDDM_MCUF1RCErrCFS_flg] -> "MCU_Fr Signal Error "/3(VDDM_MCUF1RCErrCFS_flg)
  [VDDM_MCUF1NoComCFS_flg] -> "MCU_Fr Signal Error "/2(VDDM_MCUF1NoComCFS_flg)
  VINP_MCUWarnF_enum/1 -> [VINP_MCUWarnF_enum]
  VDDM_MCUF1NoComCFS_flg/1 -> [VDDM_MCUF1NoComCFS_flg]
  No_CAN_BUS_OFF/1 -> [No_CAN_BUS_OFF]
  VPMM_PowerSta_enum/1 -> [VPMM_PowerSta_enum]
  DTC_clear_request/1 -> [DTC_clear_request]
  "MCU_Fr Signal Error "/1(VDDM_FrMCUSigErrCFS_flg) -> [VDDM_FrMCUSigErrCFS_flg]
  From5/1 -> Terminator/1
  [VDDM_FrMCUSigErrCFS_flg] -> VDDM_FrMCUSigErrCFS_flg/1
  VDDM_MCUF1RCErrCFS_flg/1 -> [VDDM_MCUF1RCErrCFS_flg]
  VDDM_MCUF1CSErrCFS_flg/1 -> [VDDM_MCUF1CSErrCFS_flg]

== system ddm/DDM/DDM/VMC_DDM/MCU_Rr Signal Error ==
  task_time_s : Inport
  VDDM_MCUF1NoComCFS_flg : Inport  Port=2
  VDDM_MCUF1RCErrCFS_flg : Inport  Port=3
  VDDM_MCUF1CSErrCFS_flg : Inport  Port=4
  No_CAN_BUS_OFF : Inport  Port=5
  VPMM_PowerSta_enum : Inport  Port=6
  VINP_MCUWarnR_enum : Inport  Port=7
  DTC_clear_request : Inport  Port=8
  From5 : From  Commented=on  GotoTag=VDDM_RrMCUSigErrDFS_flg
  "MCU_Rr Signal Error " : Subsystem
  Terminator : Terminator
  VDDM_RrMCUSigErrCFS_flg : Outport
  VDDM_RrMCUSigErrDetDTC_raw32 : Outport  Port=2
  wires:
  [VDDM_RrMCUSigErrDetDTC_raw32] -> VDDM_RrMCUSigErrDetDTC_raw32/1
  "MCU_Rr Signal Error "/2(VDDM_RrMCUSigErrDetDTC_raw32) -> [VDDM_RrMCUSigErrDetDTC_raw32]
  [task_time_s] -> "MCU_Rr Signal Error "/1(task_time_s)
  task_time_s/1 -> [task_time_s]  "task_time_s"
  [DTC_clear_request] -> "MCU_Rr Signal Error "/8(DTC_clear_request)
  [VINP_MCUWarnR_enum] -> "MCU_Rr Signal Error "/7(VINP_MCUWarnR_enum)
  [VPMM_PowerSta_enum] -> "MCU_Rr Signal Error "/6(VPMM_PowerSta_enum)
  [No_CAN_BUS_OFF] -> "MCU_Rr Signal Error "/5(No_CAN_BUS_OFF)
  [VDDM_MCUF1CSErrCFS_flg] -> "MCU_Rr Signal Error "/4(VDDM_MCUF1CSErrCFS_flg)
  [VDDM_MCUF1RCErrCFS_flg] -> "MCU_Rr Signal Error "/3(VDDM_MCUF1RCErrCFS_flg)
  [VDDM_MCUF1NoComCFS_flg] -> "MCU_Rr Signal Error "/2(VDDM_MCUF1NoComCFS_flg)
  VINP_MCUWarnR_enum/1 -> [VINP_MCUWarnR_enum]
  VDDM_MCUF1NoComCFS_flg/1 -> [VDDM_MCUF1NoComCFS_flg]
  No_CAN_BUS_OFF/1 -> [No_CAN_BUS_OFF]
  VPMM_PowerSta_enum/1 -> [VPMM_PowerSta_enum]
  DTC_clear_request/1 -> [DTC_clear_request]
  "MCU_Rr Signal Error "/1(VDDM_RrMCUSigErrCFS_flg) -> [VDDM_RrMCUSigErrCFS_flg]
  From5/1 -> Terminator/1
  [VDDM_RrMCUSigErrCFS_flg] -> VDDM_RrMCUSigErrCFS_flg/1
  VDDM_MCUF1RCErrCFS_flg/1 -> [VDDM_MCUF1RCErrCFS_flg]
  VDDM_MCUF1CSErrCFS_flg/1 -> [VDDM_MCUF1CSErrCFS_flg]

== system ddm/DDM/DDM/VMC_DDM/MSA Malfunction  ==
  task_time_s : Inport
  VDDM_BMSSigErrCFS_flg : Inport  Port=2
  VDDM_FrMCUSigErrCFS_flg : Inport  Port=3
  VDDM_RrMCUSigErrCFS_flg : Inport  Port=4
  VDDM_CCUSigErrCFS_flg : Inport  Port=5
  VDDM_ZoneSCPNoComCFS_flg : Inport  Port=6
  VDDM_MCUR1NoComCFS_flg : Inport  Port=7
  VDDM_MCUR1RCErrCFS_flg : Inport  Port=8
  VDDM_MCUR1CSErrCFS_flg : Inport  Port=9
  VDDM_MCUF1NoComCFS_flg : Inport  Port=10
  VDDM_MCUF1RCErrCFS_flg : Inport  Port=11
  VDDM_MCUF1CSErrCFS_flg : Inport  Port=12
  VDDM_ESC7NoComCFS_flg : Inport  Port=13
  VDDM_ESC7RCErrCFS_flg : Inport  Port=14
  VDDM_ESC7CSErrCFS_flg : Inport  Port=15
  VDDM_ESC1NoComCFS_flg : Inport  Port=16
  VDDM_ESC1RCErrCFS_flg : Inport  Port=17
  VDDM_ESC1CSErrCFS_flg : Inport  Port=18
  VDDM_ESC5NoComCFS_flg : Inport  Port=19
  VDDM_ESC5RCErrCFS_flg : Inport  Port=20
  VDDM_ESC5CSErrCFS_flg : Inport  Port=21
  No_CAN1_BUS_OFF : Inport  Port=22
  No_CAN3_BUS_OFF : Inport  Port=23
  No_CAN4_BUS_OFF : Inport  Port=24
  VPMM_PowerSta_enum : Inport  Port=25
  VINP_ZoneSpdCtrlMode_enum : Inport  Port=26
  DTC_clear_request : Inport  Port=27
  From5 : From  Commented=on  GotoTag=VDDM_MSAMalfuncDFS_flg
  MSA Malfunction : Subsystem
  Terminator : Terminator
  VDDM_MSAMalfuncCFS_flg : Outport
  VDDM_MSAMalfuncDetDTC_raw32 : Outport  Port=2
  wires:
  [VDDM_MSAMalfuncDetDTC_raw32] -> VDDM_MSAMalfuncDetDTC_raw32/1
  MSA Malfunction/2(VDDM_MSAMalfuncDetDTC_raw32) -> [VDDM_MSAMalfuncDetDTC_raw32]
  [DTC_clear_request] -> MSA Malfunction/27(DTC_clear_request)
  [VINP_ZoneSpdCtrlMode_enum] -> MSA Malfunction/26(VINP_ZoneSpdCtrlMode_enum)
  [VPMM_PowerSta_enum] -> MSA Malfunction/25(VPMM_PowerSta_enum)
  [No_CAN4_BUS_OFF] -> MSA Malfunction/24(No_CAN4_BUS_OFF)
  [No_CAN3_BUS_OFF] -> MSA Malfunction/23(No_CAN3_BUS_OFF)
  [No_CAN1_BUS_OFF] -> MSA Malfunction/22(No_CAN1_BUS_OFF)
  [VDDM_ESC5CSErrCFS_flg] -> MSA Malfunction/21(VDDM_ESC5CSErrCFS_flg)
  [VDDM_ESC5RCErrCFS_flg] -> MSA Malfunction/20(VDDM_ESC5RCErrCFS_flg)
  [VDDM_ESC5NoComCFS_flg] -> MSA Malfunction/19(VDDM_ESC5NoComCFS_flg)
  [VDDM_ESC1CSErrCFS_flg] -> MSA Malfunction/18(VDDM_ESC1CSErrCFS_flg)
  [VDDM_ESC1RCErrCFS_flg] -> MSA Malfunction/17(VDDM_ESC1RCErrCFS_flg)
  [VDDM_ESC1NoComCFS_flg] -> MSA Malfunction/16(VDDM_ESC1NoComCFS_flg)
  [VDDM_ESC7CSErrCFS_flg] -> MSA Malfunction/15(VDDM_ESC7CSErrCFS_flg)
  [VDDM_ESC7RCErrCFS_flg] -> MSA Malfunction/14(VDDM_ESC7RCErrCFS_flg)
  [VDDM_ESC7NoComCFS_flg] -> MSA Malfunction/13(VDDM_ESC7NoComCFS_flg)
  [VDDM_MCUF1CSErrCFS_flg] -> MSA Malfunction/12(VDDM_MCUF1CSErrCFS_flg)
  [VDDM_MCUF1RCErrCFS_flg] -> MSA Malfunction/11(VDDM_MCUF1RCErrCFS_flg)
  [VDDM_MCUF1NoComCFS_flg] -> MSA Malfunction/10(VDDM_MCUF1NoComCFS_flg)
  [VDDM_MCUR1CSErrCFS_flg] -> MSA Malfunction/9(VDDM_MCUR1CSErrCFS_flg)
  [VDDM_MCUR1RCErrCFS_flg] -> MSA Malfunction/8(VDDM_MCUR1RCErrCFS_flg)
  [VDDM_MCUR1NoComCFS_flg] -> MSA Malfunction/7(VDDM_MCUR1NoComCFS_flg)
  [VDDM_ZoneSCPNoComCFS_flg] -> MSA Malfunction/6(VDDM_ZoneSCPNoComCFS_flg)
  [VDDM_CCUSigErrCFS_flg] -> MSA Malfunction/5(VDDM_CCUSigErrCFS_flg)
  [VDDM_RrMCUSigErrCFS_flg] -> MSA Malfunction/4(VDDM_RrMCUSigErrCFS_flg)
  [VDDM_FrMCUSigErrCFS_flg] -> MSA Malfunction/3(VDDM_FrMCUSigErrCFS_flg)
  [VDDM_BMSSigErrCFS_flg] -> MSA Malfunction/2(VDDM_BMSSigErrCFS_flg)
  [task_time_s] -> MSA Malfunction/1(task_time_s)
  DTC_clear_request/1 -> [DTC_clear_request]
  No_CAN4_BUS_OFF/1 -> [No_CAN4_BUS_OFF]
  No_CAN3_BUS_OFF/1 -> [No_CAN3_BUS_OFF]
  VDDM_ESC5NoComCFS_flg/1 -> [VDDM_ESC5NoComCFS_flg]
  VDDM_ESC5RCErrCFS_flg/1 -> [VDDM_ESC5RCErrCFS_flg]
  VDDM_ESC5CSErrCFS_flg/1 -> [VDDM_ESC5CSErrCFS_flg]
  VDDM_MCUR1CSErrCFS_flg/1 -> [VDDM_MCUR1CSErrCFS_flg]
  VDDM_MCUR1RCErrCFS_flg/1 -> [VDDM_MCUR1RCErrCFS_flg]
  VDDM_MCUR1NoComCFS_flg/1 -> [VDDM_MCUR1NoComCFS_flg]
  VDDM_MCUF1NoComCFS_flg/1 -> [VDDM_MCUF1NoComCFS_flg]
  VDDM_MCUF1RCErrCFS_flg/1 -> [VDDM_MCUF1RCErrCFS_flg]
  VDDM_MCUF1CSErrCFS_flg/1 -> [VDDM_MCUF1CSErrCFS_flg]
  VDDM_ESC1CSErrCFS_flg/1 -> [VDDM_ESC1CSErrCFS_flg]
  VDDM_ESC1RCErrCFS_flg/1 -> [VDDM_ESC1RCErrCFS_flg]
  VDDM_ESC1NoComCFS_flg/1 -> [VDDM_ESC1NoComCFS_flg]
  VDDM_ESC7NoComCFS_flg/1 -> [VDDM_ESC7NoComCFS_flg]
  VDDM_ESC7RCErrCFS_flg/1 -> [VDDM_ESC7RCErrCFS_flg]
  VDDM_ESC7CSErrCFS_flg/1 -> [VDDM_ESC7CSErrCFS_flg]
  VDDM_ZoneSCPNoComCFS_flg/1 -> [VDDM_ZoneSCPNoComCFS_flg]
  VDDM_CCUSigErrCFS_flg/1 -> [VDDM_CCUSigErrCFS_flg]
  VDDM_RrMCUSigErrCFS_flg/1 -> [VDDM_RrMCUSigErrCFS_flg]
  VDDM_FrMCUSigErrCFS_flg/1 -> [VDDM_FrMCUSigErrCFS_flg]
  task_time_s/1 -> [task_time_s]  "task_time_s"
  VINP_ZoneSpdCtrlMode_enum/1 -> [VINP_ZoneSpdCtrlMode_enum]
  No_CAN1_BUS_OFF/1 -> [No_CAN1_BUS_OFF]
  VPMM_PowerSta_enum/1 -> [VPMM_PowerSta_enum]
  MSA Malfunction/1(VDDM_MSAMalfuncCFS_flg) -> [VDDM_MSAMalfuncCFS_flg]
  From5/1 -> Terminator/1
  [VDDM_MSAMalfuncCFS_flg] -> VDDM_MSAMalfuncCFS_flg/1
  VDDM_BMSSigErrCFS_flg/1 -> [VDDM_BMSSigErrCFS_flg]

== system ddm/DDM/DDM/VMC_DDM/ZoneSCP ==
  task_time_s : Inport
  VDDM_ZoneSCPNoCom_flg : Inport  Port=2
  No_CAN_BUS_OFF : Inport  Port=3
  VPMM_PowerSta_enum : Inport  Port=4
  VINP_VehSpeed_kph : Inport  Port=5
  DTC_clear_request : Inport  Port=6
  From30 : From  Commented=on  GotoTag=VDDM_VCUACCErr_flg
  Terminator : Terminator
  ZoneSCP Lost Com : Subsystem
  VDDM_ZoneSCPNoComDFS_flg : Outport
  VDDM_ZoneSCPNoComCFS_flg : Outport  Port=2
  VDDM_ZoneSCPNoComDTC_raw32 : Outport  Port=3
  wires:
  [VDDM_ZoneSCPNoComDTC_raw32] -> VDDM_ZoneSCPNoComDTC_raw32/1
  ZoneSCP Lost Com/3(VDDM_ZoneSCPNoComDTC_raw32) -> [VDDM_ZoneSCPNoComDTC_raw32]
  task_time_s/1 -> [task_time_s]  "task_time_s"
  [task_time_s] -> ZoneSCP Lost Com/1(task_time_s)
  From30/1 -> Terminator/1
  [VDDM_ZoneSCPNoComCFS_flg] -> VDDM_ZoneSCPNoComCFS_flg/1
  [VDDM_ZoneSCPNoComDFS_flg] -> VDDM_ZoneSCPNoComDFS_flg/1
  ZoneSCP Lost Com/1(VDDM_ZoneSCPNoComDFS_flg) -> [VDDM_ZoneSCPNoComDFS_flg]
  ZoneSCP Lost Com/2(VDDM_ZoneSCPNoComCFS_flg) -> [VDDM_ZoneSCPNoComCFS_flg]
  [DTC_clear_request] -> ZoneSCP Lost Com/6(DTC_clear_request)
  [VINP_VehSpeed_kph] -> ZoneSCP Lost Com/5(VINP_VehSpeed_kph)
  [VPMM_PowerSta_enum] -> ZoneSCP Lost Com/4(VPMM_PowerSta_enum)
  [No_CAN_BUS_OFF] -> ZoneSCP Lost Com/3(No_CAN_BUS_OFF)
  DTC_clear_request/1 -> [DTC_clear_request]
  VINP_VehSpeed_kph/1 -> [VINP_VehSpeed_kph]
  VPMM_PowerSta_enum/1 -> [VPMM_PowerSta_enum]
  No_CAN_BUS_OFF/1 -> [No_CAN_BUS_OFF]
  [VDDM_ZoneSCPNoCom_flg] -> ZoneSCP Lost Com/2(VDDM_ZoneSCPNoCom_flg)
  VDDM_ZoneSCPNoCom_flg/1 -> [VDDM_ZoneSCPNoCom_flg]

== system ddm/DDM/DDM/PMM/Brake switch signal abnormal/Brake switch signal abnormal ==
  note: Diagnostics and Fault Handling
  note: Test Pass Criteria
  note: Fail Safe Operation After Failure Decision
  note: Release Condition After Failure Decision
  note: Fail Safe Operation During Failure Detection
  note: Test Detection Criteria
  note: Release Condition During Failure Detection
  task_time_s : Inport
  VPMM_PowerSta_enum : Inport  Port=2
  VPMM_PwrStaSW_enum : Inport  Port=3
  BrkSWErr : Inport  Port=4
  BrkSWPass : Inport  Port=5
  DTC_clear_request : Inport  Port=6
  Constant11 : Constant  Value=KDDM_BrkSWErrPassSW_flg
  Constant15 : Constant  Value=KDDM_BrkSWErrCFSSW_flg
  Constant16 : Constant  Value=TRUE
  Constant19 : Constant  Value=ENUM_POWERSTA_OFF
  Constant{2,21,25,27} (4 alike) : Constant  Value=FALSE
  Constant20 : Constant  Value=KDDM_BrkSWErrDFSSW_flg
  Constant22 : Constant  Value=ENUM_PWRSTASW_ON
  Constant23 : Constant  Value=TRUE
  Constant24 : Constant  Value=TRUE
  Constant26 : Constant  Value=ENUM_PWRSTASW_READY
  Constant28 : Constant  Value=ENUM_PWRSTASW_ON
  Constant29 : Constant  Value=ENUM_PWRSTASW_ONHVCHRG
  Constant3 : Constant  Value=ENUM_PWRSTASW_READY
  Constant38 : Constant  Value=KDDM_BrkSWErrDetTO_s
  Constant39 : Constant  Value=ENUM_PWRSTASW_ONHVCHRG
  Constant4 : Constant  Value=KDDM_BrkSWErrPassTO_s
  Constant40 : Constant  Value=KDDM_BrkSWErrDTC_cnt
  Constant43 : Constant  Value=KDDM_BrkSWErrPassTO_s
  Constant44 : Constant  Value=KDDM_BrkSWErrDetSW_flg
  Constant5 : Constant  Value=KDDM_BrkSWErrDTC_cnt
  DTC_Couter : hcu_lib/Basic_Blocks/DTC_Couter
  DTC_Info : hcu_lib/Basic_Blocks/DTC_Info
  Data Type Conversion1 : DataTypeConversion  OutDataTypeStr=uint8
  Equal{,2,4..6,17..18} (7 alike) : RelationalOperator  Operator===  OutDataTypeStr=boolean  RndMeth=Simplest
  Equal3 : RelationalOperator  OutDataTypeStr=boolean  RndMeth=Simplest
  Logical Operator1 : Logic  Operator=NOT  AllPortsSameDT=off  OutDataTypeStr=boolean
  Logical Operator12 : Logic  AllPortsSameDT=off  OutDataTypeStr=boolean
  Logical Operator15 : Logic  AllPortsSameDT=off  OutDataTypeStr=boolean
  Logical Operator18 : Logic  AllPortsSameDT=off  OutDataTypeStr=boolean
  Logical Operator19 : Logic  Inputs=3  AllPortsSameDT=off  OutDataTypeStr=boolean
  Logical Operator2 : Logic  Operator=OR  Inputs=3  AllPortsSameDT=off  OutDataTypeStr=boolean
  Logical Operator3 : Logic  Operator=OR  Inputs=3  AllPortsSameDT=off  OutDataTypeStr=boolean
  Logical Operator4 : Logic  Operator=OR  AllPortsSameDT=off  OutDataTypeStr=boolean
  Logical Operator5 : Logic  Operator=OR  Inputs=3  AllPortsSameDT=off  OutDataTypeStr=boolean
  Logical Operator6 : Logic  Operator=NOT  AllPortsSameDT=off  OutDataTypeStr=boolean
  Logical Operator7 : Logic  Operator=OR  AllPortsSameDT=off  OutDataTypeStr=boolean
  Logical Operator8 : Logic  Operator=OR  AllPortsSameDT=off  OutDataTypeStr=boolean
  Relay : Relay  OnSwitchValue=ONE_INT  OffSwitchValue=ZERO_INT
  SR_Latch1 : Subsystem  mask(SR_Latch){}
      mask help: SR latch function.
  SR_Latch3 : hcu_lib/Basic_Blocks/SR_Latch
  SR_Latch4 : hcu_lib/Basic_Blocks/SR_Latch
  Switch{,2,4..6} (5 alike) : Switch  Criteria=u2 ~= 0
  Test Detection Criteria : hcu_lib/Basic_Blocks/Test Detection Criteria
  Timer1 : hcu_lib/Basic_Blocks/Timer
  VDDM_BrkSWErrDTC_raw32 : Outport
  VDDM_EDriveSysErrBrake_flg : Outport  Port=2
  wires:
  [VDDM_BrkSWErrCFS_flg] -> Logical Operator7/1
  Logical Operator15/1 -> DTC_Couter/2
  DTC_Couter/2 -> Data Type Conversion1/1
  Logical Operator19/1 -> DTC_Couter/1
  Relay/1 -> SR_Latch3/1
  Constant11/1 -> Logical Operator15/2
  [VDDM_BrkSWErrPass_flg] -> Logical Operator3/1
  DTC_Couter/1 -> SR_Latch4/1
  Logical Operator12/1 -> [VDDM_BrkSWErrDFS_flg]  "VDDM_BrkSWErrDFS_flg"
  Logical Operator7/1 -> SR_Latch3/2
  [VDDM_BrkSWErrCFSRls_flg] -> Logical Operator3/2
  [VDDM_BrkSWErrDet_flg] -> Logical Operator19/1
  Logical Operator3/1 -> Logical Operator15/1
  Constant44/1 -> Logical Operator19/2
  [VDDM_BrkSWErrDTC_cnt] -> Relay/1
  Data Type Conversion1/1 -> [VDDM_BrkSWErrDTC_cnt]  "VDDM_BrkSWErrDTC_cnt"
  Logical Operator4/1 -> SR_Latch4/2
  [DTC_clear_request] -> Logical Operator4/2
  Logical Operator1/1 -> Logical Operator19/3
  [DTC_clear_request] -> Logical Operator1/1
  Constant15/1 -> Logical Operator18/2
  SR_Latch4/1 -> Logical Operator18/1
  [VDDM_BrkSWErrCFSRls_flg] -> Logical Operator4/1
  Logical Operator18/1 -> [VDDM_BrkSWErrCFS_flg]  "VDDM_BrkSWErrCFS_flg"
  [DTC_clear_request] -> Logical Operator7/2
  Constant5/1 -> DTC_Couter/3
  SR_Latch3/1 -> Logical Operator12/2
  [DTC_clear_request] -> Logical Operator3/3
  Constant20/1 -> Logical Operator12/1
  Constant2/1 -> Switch6/1
  Switch5/1 -> Switch6/3
  Switch6/1 -> Test Detection Criteria/1
  [DTC_clear_request] -> Switch6/2
  [DTC_clear_request] -> DTC_Info/4
  Constant38/1 -> Test Detection Criteria/4
  [VDDM_BrkSWErrDet_flg] -> DTC_Info/1
  BrkSWPass/1 -> Switch2/1
  BrkSWErr/1 -> Switch5/1
  [VDDM_BrkSWErrCFS_flg] -> DTC_Info/3
  [VDDM_BrkSWErrPass_flg] -> DTC_Info/2
  DTC_Info/1 -> VDDM_BrkSWErrDTC_raw32/1  "VDDM_BrkSWErrDTC_raw32"
  [task_time_s] -> Timer1/3
  DTC_clear_request/1 -> [DTC_clear_request]
  [VDDM_EDriveSysErrBrake_flg] -> VDDM_EDriveSysErrBrake_flg/1
  Constant4/1 -> Equal3/2
  Logical Operator5/1 -> Switch2/2
  [VPMM_PwrStaSW_enum] -> Equal2/1
  [VPMM_PwrStaSW_enum] -> Equal17/1
  Equal18/1 -> Logical Operator5/3
  Constant3/1 -> Equal2/2
  [VPMM_PwrStaSW_enum] -> Equal18/1
  Equal2/1 -> Logical Operator5/2
  Constant39/1 -> Equal18/2
  Constant22/1 -> Equal17/2
  Equal17/1 -> Logical Operator5/1
  Constant29/1 -> Equal6/2
  Constant28/1 -> Equal5/2
  Equal6/1 -> Logical Operator2/3
  [VPMM_PwrStaSW_enum] -> Equal6/1
  Equal5/1 -> Logical Operator2/1
  [VPMM_PwrStaSW_enum] -> Equal5/1
  [task_time_s] -> Test Detection Criteria/2
  Timer1/1 -> Equal3/1
  Constant21/1 -> Switch/3
  Test Detection Criteria/1 -> [VDDM_BrkSWErrDet_flg]  "VDDM_BrkSWErrDet_flg"
  [VDDM_BrkSWErrCFS_flg] -> Switch/2
  Constant23/1 -> Switch2/3
  Constant27/1 -> Switch5/3
  Logical Operator8/1 -> Switch4/2
  Equal4/1 -> Logical Operator8/1
  Constant26/1 -> Equal/2
  Constant40/1 -> Test Detection Criteria/3
  [DTC_clear_request] -> Logical Operator8/2
  Constant25/1 -> Switch4/3
  Constant16/1 -> Switch/1
  Equal3/1 -> SR_Latch1/1(set)
  Switch/1 -> [VDDM_EDriveSysErrBrake_flg]
  SR_Latch1/1(latched) -> [VDDM_BrkSWErrPass_flg]  "VDDM_BrkSWErrPass_flg"
  Constant19/1 -> Equal4/2
  Switch4/1 -> [VDDM_BrkSWErrCFSRls_flg]  "VDDM_BrkSWErrCFSRls_flg"
  Constant43/1 -> Timer1/4
  Switch2/1 -> Timer1/1, Logical Operator6/1, SR_Latch1/2(reset)
  Constant24/1 -> Switch4/1
  Logical Operator2/1 -> Switch5/2
  Equal/1 -> Logical Operator2/2
  [VPMM_PowerSta_enum] -> Equal4/1
  [VPMM_PwrStaSW_enum] -> Equal/1
  task_time_s/1 -> [task_time_s]
  VPMM_PwrStaSW_enum/1 -> [VPMM_PwrStaSW_enum]
  VPMM_PowerSta_enum/1 -> [VPMM_PowerSta_enum]
  Logical Operator6/1 -> Timer1/2
